simulink model "NE_Red_Rooster_Delta_B"  (R2016b)
settings: Solver=FixedStepAuto  StartTime=0.0  StopTime=inf  FixedStep=0.001  RelTol=1e-3
PreLoadFcn:
  | waijung.modelPreload; % Required for working with Waijung Blockset. Do not remove.
undefined symbols (not defined in the file): ARM, DiscIntNeverNeededParam, HSEOSC, Link, LQFP100, MDK, ST, STM32F407VG
libraries: simulink x20, stm32f4_io_lib x5, stm32f4_i2c_lib x4, stm32f4_reset_lib x1, stm32f4_device_config_lib x1
(part 2 of 3)

== system NE_Red_Rooster_Delta_B/Chart/sendpwm ==
  f : TriggerPort  TriggerType=function-call  VariantControl=Variant
      settings: CopyFcn=Stateflow.SLINSF.SimulinkMan.removeBlockPreDeleteFcn  PreDeleteFcn=Stateflow.SLINSF.SimulinkMan.unsafePredeleteFcn
  Data Store Read : DataStoreRead  DataStoreName=Left_Elevon
  Data Store Read1 : DataStoreRead  DataStoreName=Right_Elevon
  Data Store Read2 : DataStoreRead  DataStoreName=Throttle_Duty
  UART Tx3 : S-Function  Priority=1  FunctionName=stm32f4_usart  Parameters=configuration,uartmodule,transfer,baudrate,inputtype,outputtype,confstr,binheaderarray,binterminatorarray,asciiheader,asciiterminator,bindatalength,packetmode,varname,sampletime,sampletimestr,blockid  SFunctionDeploymentMode=off  EnableBusSupport=off  mask(stm32f4_usart){configuration=Tx, uartmodule=2, baudrate=115200, databits=8, parity=No, stopbit=1, remaptxpin=Not used, remaprxpin=Not used, flowcontrol=None, remapctspin=Not used, remaprtspin=Not used, advanceoptions=off, rxbuffersize=512, txbuffersize=512, transfer=Non-Blocking, packetmode=Binary, binheader='4F', binterminator='2E', porttype_double=0, porttype_single=3, porttype_int8=0, porttype_uint8=0, porttype_int16=0, porttype_uint16=0, porttype_int32=0, porttype_uint32=0, asciiformat='LE=%f, RE=%f, T=%f', rx_asciiterminator=CRLF (0x0D 0x0A - "\r\n"), tx_asciiterminator=CRLF (0x0D 0x0A - "\r\n"), storagename=<empty>, varname=, inputtype=[3  1 1 1], outputtype=[0], binheaderarray=[1 79], binterminatorarray=[1 46], bindatalength=12, asciiheader='LE=%f, RE=%f, T=%f\r\n', asciiterminator=[2 13 10], sampletime=-1, sampletimestr=-1, blockid=ChartsendpwmUARTTx3, confstr=[ "dummy", "0", "*", "*", "0", "*", "*", "0", "*", "*", "0", "*", "*", "1", "4", "6", "1", "4", "5", "512", "512", "1", "2", "115200", "8", "No", "1", "None", "USART2"], lastmodule=1}
      mask prompts: uartmodule "UART Module"; baudrate "Baud rate (bps)"; databits "Data bits"; stopbit "Stop bit"; remaptxpin "Tx Pin"; remaprxpin "Rx Pin"; flowcontrol "Hardware flow control"; remapctspin "HW Flow control, CTS Pin"; remaprtspin "HW Flow control, RTS Pin"; advanceoptions "Advance options"; rxbuffersize "Rx buffer size (bytes)"; txbuffersize "Tx buffer size (bytes)"; packetmode "Packet mode"; binheader "Binary header (example: '7E 7E')"; binterminator "Binary terminator (example: '03 03')"; porttype_double "Number of data port, type DOUBLE"; porttype_single "Number of data port, type SINGLE"; porttype_int8 "Number of data port, type INT8"; porttype_uint8 "Number of data port, type UINT8"; porttype_int16 "Number of data port, type INT16"; porttype_uint16 "Number of data port, type UINT16"; porttype_int32 "Number of data port, type INT32"; porttype_uint32 "Number of data port, type UINT32"; asciiformat "Ascii format"; rx_asciiterminator "End of packet"; tx_asciiterminator "End of packet"; storagename "Buffer"; varname "Var name"; inputtype "Input data type"; outputtype "Output data type"; binheaderarray "Binary header"; binterminatorarray "Binary terminator"; bindatalength "Binary data length"; asciiheader "Ascii header (printf format)"; asciiterminator "Ascii terminator"; sampletime "Sample time (sec)"; sampletimestr "Compiled sample time (sec) in string"; confstr "Configuration string"; lastmodule "Last module selected"
      mask help:
      | Data type for Ascii format
      | %u, %i, %d, %o, %x: uint32
      | %e, %g, %f: single
      | %c: int8
      mask init:
      | stm32f4_usart_callback('init');
      mask Help: web(fullfile(waijungdocroot,'stm32f4_usart_tx.htm'), '-browser')
      mask TypeOptions configuration: Setup | Tx | Rx
      mask Callback configuration: stm32f4_usart_callback('configuration');
      mask TypeOptions uartmodule: 1 | 2 | 3 | 4 | 5 | 6
      mask Callback uartmodule: stm32f4_usart_callback('uartmodule');
      mask Callback baudrate: stm32f4_usart_callback('baudrate');
      mask TypeOptions databits: 8
      mask TypeOptions parity: No | Odd | Even
      mask TypeOptions stopbit: 0.5 | 1 | 1.5 | 2
      mask TypeOptions remaptxpin: Not used | A9 | B6
      mask TypeOptions remaprxpin: Not used | A10 | B7
      mask TypeOptions flowcontrol: None | RTS | CTS | RTS/CTS
      mask Callback flowcontrol: stm32f4_usart_callback('flowcontrol');
      mask TypeOptions remapctspin: Not used | A11
      mask TypeOptions remaprtspin: Not used | A12
      mask Callback advanceoptions: stm32f4_usart_callback('advanceoptions');
      mask TypeOptions rxbuffersize: 16 | 32 | 64 | 128 | 256 | 512 | 1024 | 2048
      mask TypeOptions txbuffersize: 16 | 32 | 64 | 128 | 256 | 512 | 1024 | 2048
      mask TypeOptions transfer: Blocking | Non-Blocking
      mask Callback transfer: stm32f4_usart_callback('transfer');
      mask TypeOptions packetmode: Ascii | Binary | Binary Vector | String Buffer | Raw Buffer
      mask Callback packetmode: stm32f4_usart_callback('packetmode');
      mask Callback binheader: stm32f4_usart_callback('binheader');
      mask Callback binterminator: stm32f4_usart_callback('binterminator');
      mask Callback porttype_double: stm32f4_usart_callback('porttype');
      mask Callback porttype_single: stm32f4_usart_callback('porttype');
      mask Callback porttype_int8: stm32f4_usart_callback('porttype');
      mask Callback porttype_uint8: stm32f4_usart_callback('porttype');
      mask Callback porttype_int16: stm32f4_usart_callback('porttype');
      mask Callback porttype_uint16: stm32f4_usart_callback('porttype');
      mask Callback porttype_int32: stm32f4_usart_callback('porttype');
      mask Callback porttype_uint32: stm32f4_usart_callback('porttype');
      mask Callback asciiformat: stm32f4_usart_callback('asciiformat');
      mask TypeOptions rx_asciiterminator: CR (0x0D - "\r") | LF (0x0A - "\n") | CRLF (0x0D 0x0A - "\r\n")
      mask Callback rx_asciiterminator: stm32f4_usart_callback('rx_asciiterminator');
      mask TypeOptions tx_asciiterminator: CR (0x0D - "\r") | LF (0x0A - "\n") | CRLF (0x0D 0x0A - "\r\n") | None
      mask Callback tx_asciiterminator: stm32f4_usart_callback('tx_asciiterminator');
      mask TypeOptions storagename: <empty>
      mask Callback storagename: stm32f4_usart_callback('storagename');
      mask Callback varname: stm32f4_usart_callback('varname');
      mask Callback sampletime: stm32f4_usart_callback('sampletime');
      mask Callback sampletimestr: stm32f4_usart_callback('sampletimestr');
      mask Callback blockid: stm32f4_usart_callback('blockid');
      mask Display: text(0.5, 0.5, 'Module: USART2_Tx\nPacket: Binary\nTransfer: Non-Blocking\nTs (sec): -1','ver','middle','hor','center'); port_label('input', 1,'single'); port_label('input', 2,'single'); port_label('input', 3,'single');
  wires:
  Data Store Read2/1 -> UART Tx3/3
  Data Store Read1/1 -> UART Tx3/2
  Data Store Read/1 -> UART Tx3/1

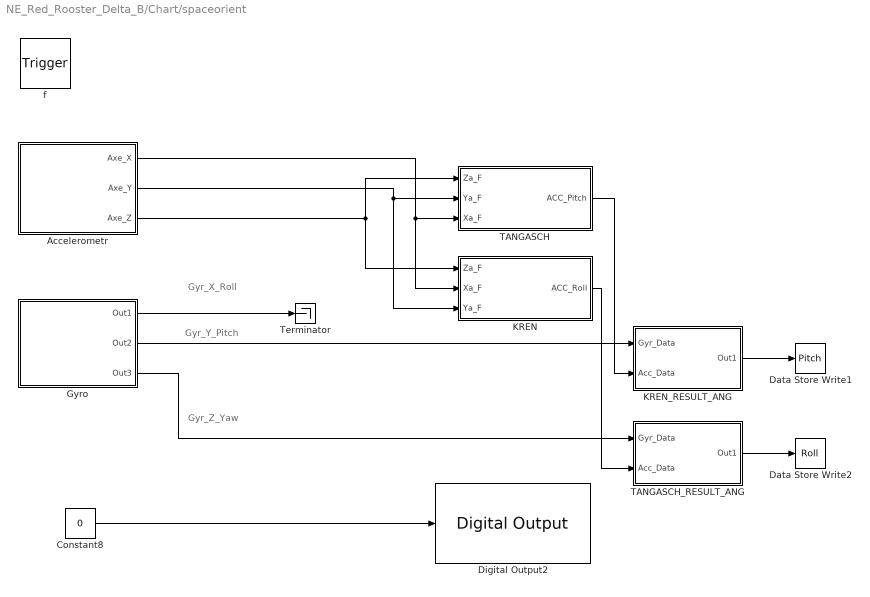
== system NE_Red_Rooster_Delta_B/Chart/spaceorient ==
  note: Gyr_X_Roll
  note: Gyr_Y_Pitch
  note: Gyr_Z_Yaw
  f : TriggerPort  TriggerType=function-call  VariantControl=Variant
      settings: CopyFcn=Stateflow.SLINSF.SimulinkMan.removeBlockPreDeleteFcn  PreDeleteFcn=Stateflow.SLINSF.SimulinkMan.unsafePredeleteFcn
  Accelerometr : Subsystem
      mask Display: image('ADXL345-1.jpg');
  Constant8 : Constant  Value=0
  Data Store Write1 : DataStoreWrite  DataStoreName=Pitch
  Data Store Write2 : DataStoreWrite  DataStoreName=Roll
  Digital Output2 : stm32f4_io_lib/Digital Output  use_bitband=on  port=D  speed=100  porttype=Push Pull  porttypestr=PP  use_pin0=off  use_pin1=off  use_pin2=off  use_pin3=off  use_pin4=off  use_pin5=off  use_pin6=off  use_pin7=off  use_pin8=off  use_pin9=off  use_pin10=off  use_pin11=off  use_pin12=off  use_pin13=off  use_pin14=off  use_pin15=on  pinstr=GPIO_Pin_15  usedpinarray="[0  0  0  0  0  0  0  0  0  0  0  0  0  0  0  1]"  bitbandingstr="#define ChartspaceorientDigitalOutput2_D15 Peripheral_BB(GPIOD->ODR, 15)  /* Output pin */"  sampletime=-1  sampletimestr=Inf  blockid=ChartspaceorientDigitalOutput2  enablecustomportlabel=off  globalinit=on  cinputportlabel=In1, In2  coutputportlabel=0
  Gyro : Subsystem
      mask Display: image('L3GD20H.jpg');
  KREN : Subsystem
  KREN_RESULT_ANG : Subsystem
  TANGASCH : Subsystem
  TANGASCH_RESULT_ANG : Subsystem
  Terminator : Terminator
  wires:
  Gyro/1(Out1) -> Terminator/1
  Accelerometr/1(Axe_X) -> TANGASCH/3(Xa_F), KREN/2(Xa_F)
  Accelerometr/2(Axe_Y) -> KREN/3(Ya_F), TANGASCH/2(Ya_F)
  Accelerometr/3(Axe_Z) -> KREN/1(Za_F), TANGASCH/1(Za_F)
  Gyro/3(Out3) -> TANGASCH_RESULT_ANG/1(Gyr_Data)
  Gyro/2(Out2) -> KREN_RESULT_ANG/1(Gyr_Data)
  TANGASCH/1(ACC_Pitch) -> KREN_RESULT_ANG/2(Acc_Data)
  KREN/1(ACC_Roll) -> TANGASCH_RESULT_ANG/2(Acc_Data)
  KREN_RESULT_ANG/1(Out1) -> Data Store Write1/1
  TANGASCH_RESULT_ANG/1(Out1) -> Data Store Write2/1
  Constant8/1 -> Digital Output2/1

== system NE_Red_Rooster_Delta_B/Reset_Subsystem ==
  Compare To Constant : simulink/Logic and Bit Operations/Compare To Constant  relop===  const=1.0  OutDataTypeStr=boolean
  Digital Input : stm32f4_io_lib/Digital Input  port=A  speed=100  porttype=None  porttypestr=NOPULL  use_pin0=on  use_pin1=off  use_pin2=off  use_pin3=off  use_pin4=off  use_pin5=off  use_pin6=off  use_pin7=off  use_pin8=off  use_pin9=off  use_pin10=off  use_pin11=off  use_pin12=off  use_pin13=off  use_pin14=off  use_pin15=off  pinstr=GPIO_Pin_0  usedpinarray="[1  0  0  0  0  0  0  0  0  0  0  0  0  0  0  0]"  bitbandingstr="#define Reset_SubsystemDigitalInput_A0 Peripheral_BB(GPIOA->IDR, 0)  /* Output pin */"  sampletime=-1  sampletimestr=0.01  blockid=Reset_SubsystemDigitalInput  enablecustomportlabel=off  glabalinit=off  cinputportlabel=In1, In2  coutputportlabel=Out1, Out2
  Enabled Subsystem : Subsystem  TreatAsAtomicUnit=on
  wires:
  Compare To Constant/1 -> Enabled Subsystem/Enable
  Digital Input/1 -> Compare To Constant/1

== system NE_Red_Rooster_Delta_B/Chart/initaccel/Init_ADXL345 ==
  Enable : EnablePort
  Compare To Zero : simulink/Logic and Bit Operations/Compare To Zero  relop===  OutDataTypeStr=boolean
  Constant : Constant  Value=0
  Constant1 : Constant  Value=hex2dec('A6')  OutDataTypeStr=uint8  SampleTime=-1
  Constant8 : Constant  Value=hex2dec('2D')  OutDataTypeStr=uint8  SampleTime=-1
  Constant9 : Constant  Value=hex2dec('08')  OutDataTypeStr=uint8  SampleTime=-1
  Data Store Write : DataStoreWrite  DataStoreName=Init_ADXL
  Digital Output1 : stm32f4_io_lib/Digital Output  use_bitband=on  port=D  speed=100  porttype=Push Pull  porttypestr=PP  use_pin0=off  use_pin1=off  use_pin2=off  use_pin3=off  use_pin4=off  use_pin5=off  use_pin6=off  use_pin7=off  use_pin8=off  use_pin9=off  use_pin10=off  use_pin11=off  use_pin12=off  use_pin13=on  use_pin14=off  use_pin15=off  pinstr=GPIO_Pin_13  usedpinarray="[0  0  0  0  0  0  0  0  0  0  0  0  0  1  0  0]"  bitbandingstr="#define ChartinitaccelInit_ADXL345DigitalOutput1_D13 Peripheral_BB(GPIOD->ODR, 13)  /* Output pin */"  sampletime=-1  sampletimestr=Inf  blockid=ChartinitaccelInit_ADXL345DigitalOutput1  enablecustomportlabel=off  globalinit=off  cinputportlabel=In1, In2  coutputportlabel=0
  I2C Master Read/Write1 : stm32f4_i2c_lib/I2C Master Read//Write  configuration=Transaction  module=1  lastmodule=3  transfer=Blocking  dutycycle=TLow/THigh = 2  clkspeed=400  timeout=25  writecount=2  readcount=0  sdapin=C9  sclpin=A8  waitwritetime=0  forcestop=off  inputtypearray=[3 3 3 3]  outputtypearray=[1 3]  confstr="[\"C\",\"9\",\"A\",\"8\",\"1\",\"1\",\"6\",\"0\",\"I2C_DutyCycle_2\",\"0\",\"off\"]"  sampletime=-1  sampletimestr=-1  blockid=ChartinitaccelInit_ADXL345I2CMasterReadWrite1
  Subsystem : Subsystem
  Terminator : Terminator
  wires:
  Constant9/1 -> I2C Master Read/Write1/3
  I2C Master Read/Write1/1 -> Compare To Zero/1
  Constant1/1 -> I2C Master Read/Write1/1
  Constant8/1 -> I2C Master Read/Write1/2
  Compare To Zero/1 -> Subsystem/Enable
  Subsystem/1(Out1) -> Terminator/1
  Constant/1 -> Digital Output1/1, Data Store Write/1

== system NE_Red_Rooster_Delta_B/Chart/initgyro/Init_L3GD4200  ==
  Enable : EnablePort
  Compare To Zero : simulink/Logic and Bit Operations/Compare To Zero  relop===  OutDataTypeStr=boolean  ZeroCross=off
  Constant : Constant  Value=0
  Data Store Write : DataStoreWrite  DataStoreName=Init_L3GD
  Get Init L3G4200D1 : Subsystem
  Init L3G4200D : Subsystem  TreatAsAtomicUnit=on
  SlvAddr1 : Constant  Value=hex2dec('D2')  OutDataTypeStr=uint8  SampleTime=-1
  wires:
  Compare To Zero/1 -> Init L3G4200D/Enable
  Get Init L3G4200D1/1(Initial Done) -> Compare To Zero/1
  SlvAddr1/1 -> Get Init L3G4200D1/1(SlvAddr)
  Constant/1 -> Data Store Write/1

== system NE_Red_Rooster_Delta_B/Chart/pwm/If Action Subsystem ==
  In1 : Inport
  In2 : Inport  Port=2
  In3 : Inport  Port=3
  Action Port : ActionPort  ActionType=then
  Out1 : Outport
  Out2 : Outport  Port=2
  Out3 : Outport  Port=3
  wires:
  In1/1 -> Out1/1
  In2/1 -> Out2/1
  In3/1 -> Out3/1

== system NE_Red_Rooster_Delta_B/Chart/pwm/If Action Subsystem1 ==
  In1 : Inport
  In2 : Inport  Port=2
  In3 : Inport  Port=3
  Action Port : ActionPort  ActionType=then
  Out1 : Outport
  Out2 : Outport  Port=2
  Out3 : Outport  Port=3
  wires:
  In1/1 -> Out1/1
  In2/1 -> Out2/1
  In3/1 -> Out3/1

== system NE_Red_Rooster_Delta_B/Chart/pwm/If Action Subsystem2 ==
  In1 : Inport
  In2 : Inport  Port=2
  In3 : Inport  Port=3
  Action Port : ActionPort  ActionType=then
  Out1 : Outport
  Out2 : Outport  Port=2
  Out3 : Outport  Port=3
  wires:
  In3/1 -> Out3/1
  In2/1 -> Out2/1
  In1/1 -> Out1/1

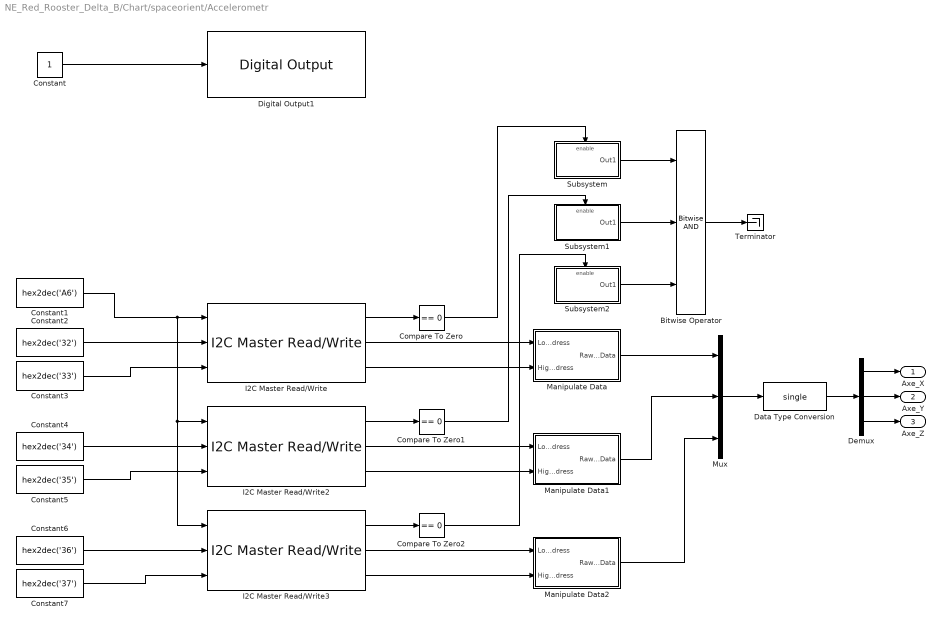
== system NE_Red_Rooster_Delta_B/Chart/spaceorient/Accelerometr ==
  Bitwise Operator : simulink/Logic and Bit Operations/Bitwise Operator  logicop=AND  UseBitMask=off  NumInputPorts=3  BitMask=bin2dec('11011001')  BitMaskRealWorld=Stored Integer
  Compare To Zero : simulink/Logic and Bit Operations/Compare To Zero  relop===  OutDataTypeStr=boolean
  Compare To Zero1 : simulink/Logic and Bit Operations/Compare To Zero  relop===  OutDataTypeStr=boolean
  Compare To Zero2 : simulink/Logic and Bit Operations/Compare To Zero  relop===  OutDataTypeStr=boolean
  Constant : Constant
  Constant1 : Constant  Value=hex2dec('A6')  OutDataTypeStr=uint8  SampleTime=-1
  Constant2 : Constant  Value=hex2dec('32')  OutDataTypeStr=uint8  SampleTime=-1
  Constant3 : Constant  Value=hex2dec('33')  OutDataTypeStr=uint8  SampleTime=-1
  Constant4 : Constant  Value=hex2dec('34')  OutDataTypeStr=uint8  SampleTime=-1
  Constant5 : Constant  Value=hex2dec('35')  OutDataTypeStr=uint8  SampleTime=-1
  Constant6 : Constant  Value=hex2dec('36')  OutDataTypeStr=uint8  SampleTime=-1
  Constant7 : Constant  Value=hex2dec('37')  OutDataTypeStr=uint8  SampleTime=-1
  Data Type Conversion : DataTypeConversion  OutDataTypeStr=single
  Demux : Demux  Outputs=3
  Digital Output1 : stm32f4_io_lib/Digital Output  use_bitband=on  port=D  speed=100  porttype=Push Pull  porttypestr=PP  use_pin0=off  use_pin1=off  use_pin2=off  use_pin3=off  use_pin4=off  use_pin5=off  use_pin6=off  use_pin7=off  use_pin8=off  use_pin9=off  use_pin10=off  use_pin11=off  use_pin12=off  use_pin13=off  use_pin14=off  use_pin15=on  pinstr=GPIO_Pin_15  usedpinarray="[0  0  0  0  0  0  0  0  0  0  0  0  0  0  0  1]"  bitbandingstr="#define ChartspaceorientAccelerometrDigitalOutput1_D15 Peripheral_BB(GPIOD->ODR, 15)  /* Output pin */"  sampletime=-1  sampletimestr=Inf  blockid=ChartspaceorientAccelerometrDigitalOutput1  enablecustomportlabel=off  globalinit=on  cinputportlabel=In1, In2  coutputportlabel=0
  I2C Master Read/Write : stm32f4_i2c_lib/I2C Master Read//Write  configuration=Transaction  module=1  lastmodule=3  transfer=Blocking  dutycycle=TLow/THigh = 2  clkspeed=400  timeout=25  writecount=2  readcount=2  sdapin=C9  sclpin=A8  waitwritetime=0  forcestop=off  inputtypearray=[3 3 3 3]  outputtypearray=[3 3 3 3]  confstr="[\"C\",\"9\",\"A\",\"8\",\"1\",\"1\",\"6\",\"0\",\"I2C_DutyCycle_2\",\"0\",\"off\"]"  sampletime=-1  sampletimestr=-1  blockid=ChartspaceorientAccelerometrI2CMasterReadWrite
  I2C Master Read/Write2 : stm32f4_i2c_lib/I2C Master Read//Write  configuration=Transaction  module=1  lastmodule=3  transfer=Blocking  dutycycle=TLow/THigh = 2  clkspeed=400  timeout=25  writecount=2  readcount=2  sdapin=C9  sclpin=A8  waitwritetime=0  forcestop=off  inputtypearray=[3 3 3 3]  outputtypearray=[3 3 3 3]  confstr="[\"C\",\"9\",\"A\",\"8\",\"1\",\"1\",\"6\",\"0\",\"I2C_DutyCycle_2\",\"0\",\"off\"]"  sampletime=-1  sampletimestr=-1  blockid=ChartspaceorientAccelerometrI2CMasterReadWrite2
  I2C Master Read/Write3 : stm32f4_i2c_lib/I2C Master Read//Write  configuration=Transaction  module=1  lastmodule=3  transfer=Blocking  dutycycle=TLow/THigh = 2  clkspeed=400  timeout=25  writecount=2  readcount=2  sdapin=C9  sclpin=A8  waitwritetime=0  forcestop=off  inputtypearray=[3 3 3 3]  outputtypearray=[3 3 3 3]  confstr="[\"C\",\"9\",\"A\",\"8\",\"1\",\"1\",\"6\",\"0\",\"I2C_DutyCycle_2\",\"0\",\"off\"]"  sampletime=-1  sampletimestr=-1  blockid=ChartspaceorientAccelerometrI2CMasterReadWrite3
  Manipulate Data : Subsystem
  Manipulate Data1 : Subsystem
  Manipulate Data2 : Subsystem
  Mux : Mux  Inputs=3
  Subsystem : Subsystem
  Subsystem1 : Subsystem
  Subsystem2 : Subsystem
  Terminator : Terminator
  Axe_X : Outport
  Axe_Y : Outport  Port=2
  Axe_Z : Outport  Port=3
  wires:
  I2C Master Read/Write3/2 -> Manipulate Data2/1(LowAddress)
  I2C Master Read/Write2/3 -> Manipulate Data1/2(HighAddress)
  I2C Master Read/Write/1 -> Compare To Zero/1
  Constant7/1 -> I2C Master Read/Write3/3
  I2C Master Read/Write3/3 -> Manipulate Data2/2(HighAddress)
  Mux/1 -> Data Type Conversion/1
  Constant4/1 -> I2C Master Read/Write2/2
  Constant1/1 -> I2C Master Read/Write3/1, I2C Master Read/Write2/1, I2C Master Read/Write/1
  I2C Master Read/Write2/2 -> Manipulate Data1/1(LowAddress)
  I2C Master Read/Write/3 -> Manipulate Data/2(HighAddress)
  I2C Master Read/Write3/1 -> Compare To Zero2/1
  Constant6/1 -> I2C Master Read/Write3/2
  Manipulate Data2/1(RawAccData) -> Mux/3
  Constant5/1 -> I2C Master Read/Write2/3
  Manipulate Data1/1(RawAccData) -> Mux/2
  I2C Master Read/Write/2 -> Manipulate Data/1(LowAddress)
  Constant2/1 -> I2C Master Read/Write/2
  Constant3/1 -> I2C Master Read/Write/3
  I2C Master Read/Write2/1 -> Compare To Zero1/1
  Manipulate Data/1(RawAccData) -> Mux/1
  Compare To Zero/1 -> Subsystem/Enable
  Compare To Zero1/1 -> Subsystem1/Enable
  Compare To Zero2/1 -> Subsystem2/Enable
  Data Type Conversion/1 -> Demux/1
  Demux/2 -> Axe_Y/1
  Demux/1 -> Axe_X/1
  Demux/3 -> Axe_Z/1
  Subsystem/1(Out1) -> Bitwise Operator/1
  Subsystem1/1(Out1) -> Bitwise Operator/2
  Subsystem2/1(Out1) -> Bitwise Operator/3
  Bitwise Operator/1 -> Terminator/1
  Constant/1 -> Digital Output1/1

== system NE_Red_Rooster_Delta_B/Chart/spaceorient/Gyro ==
  Compare To Zero1 : simulink/Logic and Bit Operations/Compare To Zero  relop===  OutDataTypeStr=boolean  ZeroCross=off
  Data_transformation : Subsystem
  L3G4200D : Subsystem
  Success : Subsystem
      mask Display: image('C:\Users\Alexander Gorbunov\Pictures\Roll_Pitch_Yaw.JPG');
  Out1 : Outport
  Out2 : Outport  Port=2
  Out3 : Outport  Port=3
  wires:
  Success/1(Gyr_X) -> Data_transformation/1(In1)
  L3G4200D/1(Status) -> Compare To Zero1/1
  L3G4200D/4(Z) -> Success/3(In3)
  L3G4200D/3(Y) -> Success/2(In2)
  Success/2(Gyr_Y) -> Data_transformation/2(In2)
  Success/3(Gyr_Z) -> Data_transformation/3(In3)
  L3G4200D/2(X) -> Success/1(In1)
  Compare To Zero1/1 -> Success/Enable
  Data_transformation/1(Out1) -> Out1/1
  Data_transformation/2(Out2) -> Out2/1
  Data_transformation/3(Out3) -> Out3/1

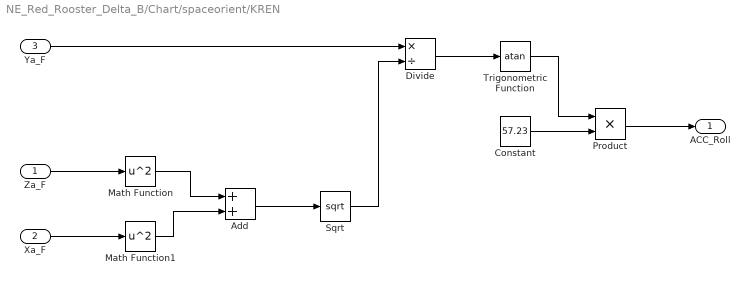
== system NE_Red_Rooster_Delta_B/Chart/spaceorient/KREN ==
  Za_F : Inport
  Xa_F : Inport  Port=2
  Ya_F : Inport  Port=3
  Add : Sum
  Constant : Constant  Value=57.23
  Divide : Product  Inputs=*/
  Math Function : Math  Operator=square  SaturateOnIntegerOverflow=on
  Math Function1 : Math  Operator=square  SaturateOnIntegerOverflow=on
  Product : Product
  Sqrt : Sqrt  SaturateOnIntegerOverflow=on
  Trigonometric Function : Trigonometry  Operator=atan
  ACC_Roll : Outport
  wires:
  Sqrt/1 -> Divide/2
  Za_F/1 -> Math Function/1
  Ya_F/1 -> Divide/1
  Xa_F/1 -> Math Function1/1
  Add/1 -> Sqrt/1
  Trigonometric Function/1 -> Product/1
  Divide/1 -> Trigonometric Function/1
  Math Function/1 -> Add/1
  Math Function1/1 -> Add/2
  Constant/1 -> Product/2
  Product/1 -> ACC_Roll/1

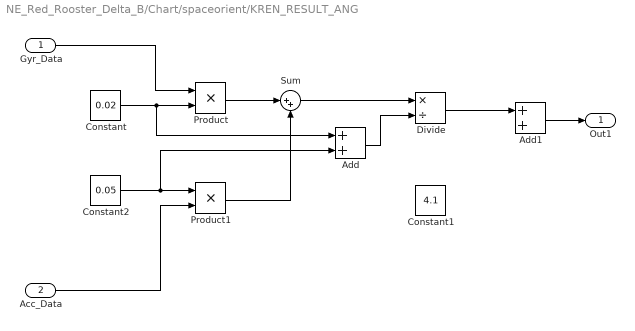
== system NE_Red_Rooster_Delta_B/Chart/spaceorient/KREN_RESULT_ANG ==
  Gyr_Data : Inport
  Acc_Data : Inport  Port=2
  Add : Sum
  Add1 : Sum
  Constant : Constant  Value=0.02
  Constant1 : Constant  Value=4.1
  Constant2 : Constant  Value=0.05
  Divide : Product  Inputs=*/
  Product : Product
  Product1 : Product
  Sum : Sum  Inputs=|++
  Out1 : Outport
  wires:
  Acc_Data/1 -> Product1/2
  Constant/1 -> Add/1, Product/2
  Product/1 -> Sum/1
  Product1/1 -> Sum/2
  Constant2/1 -> Add/2, Product1/1
  Gyr_Data/1 -> Product/1
  Sum/1 -> Divide/1
  Add/1 -> Divide/2
  Divide/1 -> Add1/1
  Add1/1 -> Out1/1

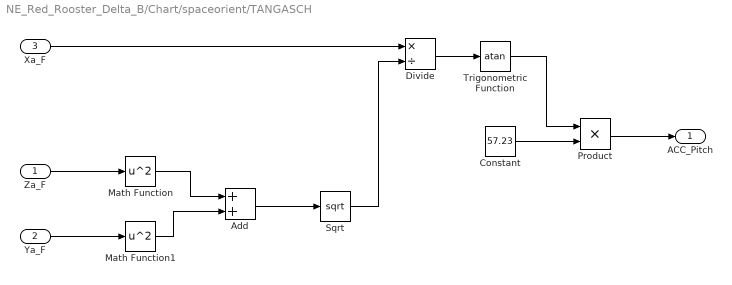
== system NE_Red_Rooster_Delta_B/Chart/spaceorient/TANGASCH ==
  Za_F : Inport
  Ya_F : Inport  Port=2
  Xa_F : Inport  Port=3
  Add : Sum
  Constant : Constant  Value=57.23
  Divide : Product  Inputs=*/
  Math Function : Math  Operator=square  SaturateOnIntegerOverflow=on
  Math Function1 : Math  Operator=square  SaturateOnIntegerOverflow=on
  Product : Product
  Sqrt : Sqrt  SaturateOnIntegerOverflow=on
  Trigonometric Function : Trigonometry  Operator=atan
  ACC_Pitch : Outport
  wires:
  Math Function1/1 -> Add/2
  Math Function/1 -> Add/1
  Divide/1 -> Trigonometric Function/1
  Trigonometric Function/1 -> Product/1
  Add/1 -> Sqrt/1
  Ya_F/1 -> Math Function1/1
  Xa_F/1 -> Divide/1
  Za_F/1 -> Math Function/1
  Sqrt/1 -> Divide/2
  Constant/1 -> Product/2
  Product/1 -> ACC_Pitch/1

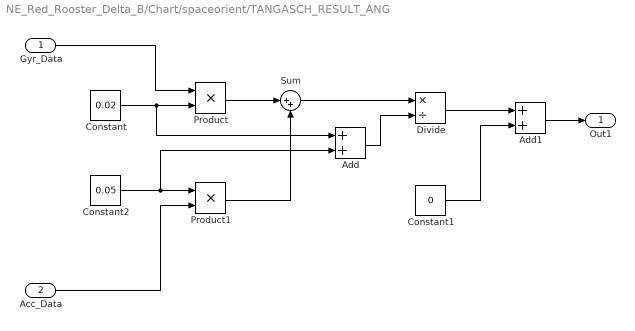
== system NE_Red_Rooster_Delta_B/Chart/spaceorient/TANGASCH_RESULT_ANG ==
  Gyr_Data : Inport
  Acc_Data : Inport  Port=2
  Add : Sum
  Add1 : Sum
  Constant : Constant  Value=0.02
  Constant1 : Constant  Value=0
  Constant2 : Constant  Value=0.05
  Divide : Product  Inputs=*/
  Product : Product
  Product1 : Product
  Sum : Sum  Inputs=|++
  Out1 : Outport
  wires:
  Constant1/1 -> Add1/2
  Add1/1 -> Out1/1
  Divide/1 -> Add1/1
  Add/1 -> Divide/2
  Sum/1 -> Divide/1
  Gyr_Data/1 -> Product/1
  Constant2/1 -> Product1/1, Add/2
  Product1/1 -> Sum/2
  Product/1 -> Sum/1
  Constant/1 -> Product/2, Add/1
  Acc_Data/1 -> Product1/2

== system NE_Red_Rooster_Delta_B/Reset_Subsystem/Enabled Subsystem ==
  Enable : EnablePort
  System Reset : stm32f4_reset_lib/System Reset  conf=<empty>  sampletime=-1  sampletimestr=0.01  blockid=Reset_SubsystemEnabledSubsystemSystemReset  inputarray=[]  inputlabelarray={}  outputarray=[]  outputlabelarray={}  compat=0  confstr="[\"Param1\",\"Param1\"]"

== system NE_Red_Rooster_Delta_B/Chart/initaccel/Init_ADXL345/Subsystem ==
  Enable : EnablePort
  Constant : Constant
  Out1 : Outport
  wires:
  Constant/1 -> Out1/1

== system NE_Red_Rooster_Delta_B/Chart/initgyro/Init_L3GD4200 /Get Init L3G4200D1 ==
  SlvAddr : Inport
  Bitwise Operator : simulink/Logic and Bit Operations/Bitwise Operator  logicop=AND  UseBitMask=off  NumInputPorts=4  BitMask=bin2dec('11011001')  BitMaskRealWorld=Stored Integer
  CNTRL_REG1 : Constant  Value=hex2dec('20')  OutDataTypeStr=uint8  SampleTime=-1
  CNTRL_REG4 : Constant  Value=hex2dec('23')  OutDataTypeStr=uint8  SampleTime=-1
  Compare To Constant : simulink/Logic and Bit Operations/Compare To Constant  relop===  const=0  OutDataTypeStr=uint8  ZeroCross=off
  Compare To Constant1 : simulink/Logic and Bit Operations/Compare To Constant  relop===  const=hex2dec('0F')  OutDataTypeStr=uint8  ZeroCross=off
  Compare To Constant2 : simulink/Logic and Bit Operations/Compare To Constant  relop===  const=0  OutDataTypeStr=uint8  ZeroCross=off
  Compare To Constant3 : simulink/Logic and Bit Operations/Compare To Constant  relop===  const=0  OutDataTypeStr=uint8  ZeroCross=off
  I2C Master Read/Write : S-Function  FunctionName=stm32f4_i2c  Parameters=configuration,module,transfer,clkspeed,timeout,sdapin,sclpin,writecount,readcount,inputtypearray,outputtypearray,confstr,sampletime,sampletimestr,blockid  SFunctionDeploymentMode=off  EnableBusSupport=off  mask(stm32f4_i2c){configuration=Transaction, module=1, lastmodule=3, transfer=Blocking, dutycycle=TLow/THigh = 2, clkspeed=400, timeout=25, writecount=1, readcount=1, sdapin=C9, sclpin=A8, waitwritetime=0, inputtypearray=[2 3 3], outputtypearray=[2 3 3], confstr=["C","9","A","8","1","1","6","0","I2C_DutyCycle_2","0","off"], sampletime=-1, sampletimestr=-1, blockid=ChartinitgyroInit_L3GD4200GetInitL3G4200D1I2CMasterReadWrite}
      mask prompts: module "I2C Module"; lastmodule "Last module"; transfer "Transfer mode"; dutycycle "Duty cycle in fast mode"; clkspeed "Clock speed (kHz)"; timeout "Timeout (ms)"; writecount "Bytes write count"; readcount "Bytes read count"; sdapin "SDA pin"; sclpin "SCL pin"; waitwritetime "Wait write time (ms), default is 0"; inputtypearray "Input type array"; outputtypearray "Output type array"; confstr "Configuration string"; sampletime "Sample time (sec)"; sampletimestr "Compiled sample time (sec) in string"
      mask init:
      | stm32f4_i2c_callback('init');
      mask Help: web(fullfile(waijungdocroot,'stm32f4_i2c.htm'), '-browser')
      mask TypeOptions configuration: Setup | Transaction
      mask Callback configuration: stm32f4_i2c_callback('configuration');
      mask TypeOptions module: 1 | 2 | 3
      mask Callback module: stm32f4_i2c_callback('module');
      mask TypeOptions transfer: Blocking | Non-blocking
      mask TypeOptions dutycycle: TLow/THigh = 16/9 | TLow/THigh = 2
      mask Callback dutycycle: stm32f4_i2c_callback('dutycycle');
      mask Callback writecount: stm32f4_i2c_callback('writecount');
      mask Callback readcount: stm32f4_i2c_callback('readcount');
      mask TypeOptions sdapin: - | C9
      mask Callback sdapin: stm32f4_i2c_callback('sdapin');
      mask TypeOptions sclpin: - | A8
      mask Callback sclpin: stm32f4_i2c_callback('sclpin');
      mask Callback confstr: stm32f4_i2c_callback('confstr');
      mask Callback sampletime: stm32f4_i2c_callback('sampletime');
      mask Callback sampletimestr: stm32f4_i2c_callback('sampletimestr');
      mask Callback blockid: stm32f4_i2c_callback('blockid');
      mask Display: text(0.5, 0.5, 'Module: I2C1\nTransfer: Blocking\nWrite: 1 bytes\nRead: 1 bytes\nTs (sec): -1','ver','middle','hor','center');port_label('input', 1,'SlvAddr');port_label('input', 2,'Wr0 (uint8)');port_label('output', 1,'Status');port_label('output', 2,'Rd0 (uint8)');
  I2C Master Read/Write1 : S-Function  FunctionName=stm32f4_i2c  Parameters=configuration,module,transfer,clkspeed,timeout,sdapin,sclpin,writecount,readcount,inputtypearray,outputtypearray,confstr,sampletime,sampletimestr,blockid  SFunctionDeploymentMode=off  EnableBusSupport=off  mask(stm32f4_i2c){configuration=Transaction, module=1, lastmodule=3, transfer=Blocking, dutycycle=TLow/THigh = 2, clkspeed=400, timeout=25, writecount=1, readcount=1, sdapin=C9, sclpin=A8, waitwritetime=0, inputtypearray=[2 3 3], outputtypearray=[2 3 3], confstr=["C","9","A","8","1","1","6","0","I2C_DutyCycle_2","0","off"], sampletime=-1, sampletimestr=-1, blockid=ChartinitgyroInit_L3GD4200GetInitL3G4200D1I2CMasterReadWrite1}
      mask prompts: module "I2C Module"; lastmodule "Last module"; transfer "Transfer mode"; dutycycle "Duty cycle in fast mode"; clkspeed "Clock speed (kHz)"; timeout "Timeout (ms)"; writecount "Bytes write count"; readcount "Bytes read count"; sdapin "SDA pin"; sclpin "SCL pin"; waitwritetime "Wait write time (ms), default is 0"; inputtypearray "Input type array"; outputtypearray "Output type array"; confstr "Configuration string"; sampletime "Sample time (sec)"; sampletimestr "Compiled sample time (sec) in string"
      mask init:
      | stm32f4_i2c_callback('init');
      mask Help: web(fullfile(waijungdocroot,'stm32f4_i2c.htm'), '-browser')
      mask TypeOptions configuration: Setup | Transaction
      mask Callback configuration: stm32f4_i2c_callback('configuration');
      mask TypeOptions module: 1 | 2 | 3
      mask Callback module: stm32f4_i2c_callback('module');
      mask TypeOptions transfer: Blocking | Non-blocking
      mask TypeOptions dutycycle: TLow/THigh = 16/9 | TLow/THigh = 2
      mask Callback dutycycle: stm32f4_i2c_callback('dutycycle');
      mask Callback writecount: stm32f4_i2c_callback('writecount');
      mask Callback readcount: stm32f4_i2c_callback('readcount');
      mask TypeOptions sdapin: - | C9
      mask Callback sdapin: stm32f4_i2c_callback('sdapin');
      mask TypeOptions sclpin: - | A8
      mask Callback sclpin: stm32f4_i2c_callback('sclpin');
      mask Callback confstr: stm32f4_i2c_callback('confstr');
      mask Callback sampletime: stm32f4_i2c_callback('sampletime');
      mask Callback sampletimestr: stm32f4_i2c_callback('sampletimestr');
      mask Callback blockid: stm32f4_i2c_callback('blockid');
      mask Display: text(0.5, 0.5, 'Module: I2C1\nTransfer: Blocking\nWrite: 1 bytes\nRead: 1 bytes\nTs (sec): -1','ver','middle','hor','center');port_label('input', 1,'SlvAddr');port_label('input', 2,'Wr0 (uint8)');port_label('output', 1,'Status');port_label('output', 2,'Rd0 (uint8)');
  Initial Done : Outport
  wires:
  Compare To Constant3/1 -> Bitwise Operator/4
  Compare To Constant2/1 -> Bitwise Operator/3
  Compare To Constant1/1 -> Bitwise Operator/2
  Compare To Constant/1 -> Bitwise Operator/1
  Bitwise Operator/1 -> Initial Done/1
  I2C Master Read/Write1/2 -> Compare To Constant3/1
  I2C Master Read/Write1/1 -> Compare To Constant2/1
  I2C Master Read/Write/2 -> Compare To Constant1/1
  I2C Master Read/Write/1 -> Compare To Constant/1
  SlvAddr/1 -> I2C Master Read/Write/1, I2C Master Read/Write1/1
  CNTRL_REG1/1 -> I2C Master Read/Write/2
  CNTRL_REG4/1 -> I2C Master Read/Write1/2

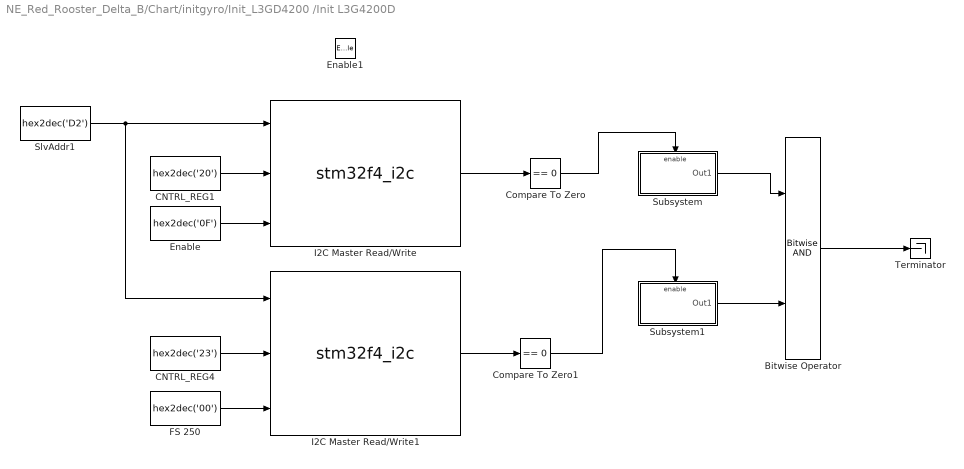
== system NE_Red_Rooster_Delta_B/Chart/initgyro/Init_L3GD4200 /Init L3G4200D ==
  Enable1 : EnablePort  PropagateVarSize=During execution
  Bitwise Operator : simulink/Logic and Bit Operations/Bitwise Operator  logicop=AND  UseBitMask=off  NumInputPorts=2  BitMask=bin2dec('11011001')  BitMaskRealWorld=Stored Integer
  CNTRL_REG1 : Constant  Value=hex2dec('20')  OutDataTypeStr=uint8  SampleTime=-1
  CNTRL_REG4 : Constant  Value=hex2dec('23')  OutDataTypeStr=uint8  SampleTime=-1
  Compare To Zero : simulink/Logic and Bit Operations/Compare To Zero  relop===  OutDataTypeStr=boolean
  Compare To Zero1 : simulink/Logic and Bit Operations/Compare To Zero  relop===  OutDataTypeStr=boolean
  Enable : Constant  Value=hex2dec('0F')  OutDataTypeStr=uint8  SampleTime=-1
  FS 250 : Constant  Value=hex2dec('00')  OutDataTypeStr=uint8  SampleTime=-1
  I2C Master Read/Write : S-Function  FunctionName=stm32f4_i2c  Parameters=configuration,module,transfer,clkspeed,timeout,sdapin,sclpin,writecount,readcount,inputtypearray,outputtypearray,confstr,sampletime,sampletimestr,blockid  SFunctionDeploymentMode=off  EnableBusSupport=off  mask(stm32f4_i2c){configuration=Transaction, module=1, lastmodule=3, transfer=Blocking, dutycycle=TLow/THigh = 2, clkspeed=400, timeout=25, writecount=2, readcount=0, sdapin=C9, sclpin=A8, waitwritetime=0, inputtypearray=[3 3 3 3], outputtypearray=[1 3], confstr=["C","9","A","8","1","1","6","0","I2C_DutyCycle_2","0","off"], sampletime=-1, sampletimestr=-1, blockid=ChartinitgyroInit_L3GD4200InitL3G4200DI2CMasterReadWrite}
      mask prompts: module "I2C Module"; lastmodule "Last module"; transfer "Transfer mode"; dutycycle "Duty cycle in fast mode"; clkspeed "Clock speed (kHz)"; timeout "Timeout (ms)"; writecount "Bytes write count"; readcount "Bytes read count"; sdapin "SDA pin"; sclpin "SCL pin"; waitwritetime "Wait write time (ms), default is 0"; inputtypearray "Input type array"; outputtypearray "Output type array"; confstr "Configuration string"; sampletime "Sample time (sec)"; sampletimestr "Compiled sample time (sec) in string"
      mask init:
      | stm32f4_i2c_callback('init');
      mask Help: web(fullfile(waijungdocroot,'stm32f4_i2c.htm'), '-browser')
      mask TypeOptions configuration: Setup | Transaction
      mask Callback configuration: stm32f4_i2c_callback('configuration');
      mask TypeOptions module: 1 | 2 | 3
      mask Callback module: stm32f4_i2c_callback('module');
      mask TypeOptions transfer: Blocking | Non-blocking
      mask TypeOptions dutycycle: TLow/THigh = 16/9 | TLow/THigh = 2
      mask Callback dutycycle: stm32f4_i2c_callback('dutycycle');
      mask Callback writecount: stm32f4_i2c_callback('writecount');
      mask Callback readcount: stm32f4_i2c_callback('readcount');
      mask TypeOptions sdapin: - | C9
      mask Callback sdapin: stm32f4_i2c_callback('sdapin');
      mask TypeOptions sclpin: - | A8
      mask Callback sclpin: stm32f4_i2c_callback('sclpin');
      mask Callback confstr: stm32f4_i2c_callback('confstr');
      mask Callback sampletime: stm32f4_i2c_callback('sampletime');
      mask Callback sampletimestr: stm32f4_i2c_callback('sampletimestr');
      mask Callback blockid: stm32f4_i2c_callback('blockid');
      mask Display: text(0.5, 0.5, 'Module: I2C1\nTransfer: Blocking\nWrite: 2 bytes\nRead: 0 bytes\nTs (sec): -1','ver','middle','hor','center');port_label('input', 1,'SlvAddr');port_label('input', 2,'Wr0 (uint8)');port_label('input', 3,'Wr1 (uint8)');port_label('output', 1,'Status');
  I2C Master Read/Write1 : S-Function  FunctionName=stm32f4_i2c  Parameters=configuration,module,transfer,clkspeed,timeout,sdapin,sclpin,writecount,readcount,inputtypearray,outputtypearray,confstr,sampletime,sampletimestr,blockid  SFunctionDeploymentMode=off  EnableBusSupport=off  mask(stm32f4_i2c){configuration=Transaction, module=1, lastmodule=3, transfer=Blocking, dutycycle=TLow/THigh = 2, clkspeed=400, timeout=25, writecount=2, readcount=0, sdapin=C9, sclpin=A8, waitwritetime=0, inputtypearray=[3 3 3 3], outputtypearray=[1 3], confstr=["C","9","A","8","1","1","6","0","I2C_DutyCycle_2","0","off"], sampletime=-1, sampletimestr=-1, blockid=ChartinitgyroInit_L3GD4200InitL3G4200DI2CMasterReadWrite1}
      mask prompts: module "I2C Module"; lastmodule "Last module"; transfer "Transfer mode"; dutycycle "Duty cycle in fast mode"; clkspeed "Clock speed (kHz)"; timeout "Timeout (ms)"; writecount "Bytes write count"; readcount "Bytes read count"; sdapin "SDA pin"; sclpin "SCL pin"; waitwritetime "Wait write time (ms), default is 0"; inputtypearray "Input type array"; outputtypearray "Output type array"; confstr "Configuration string"; sampletime "Sample time (sec)"; sampletimestr "Compiled sample time (sec) in string"
      mask init:
      | stm32f4_i2c_callback('init');
      mask Help: web(fullfile(waijungdocroot,'stm32f4_i2c.htm'), '-browser')
      mask TypeOptions configuration: Setup | Transaction
      mask Callback configuration: stm32f4_i2c_callback('configuration');
      mask TypeOptions module: 1 | 2 | 3
      mask Callback module: stm32f4_i2c_callback('module');
      mask TypeOptions transfer: Blocking | Non-blocking
      mask TypeOptions dutycycle: TLow/THigh = 16/9 | TLow/THigh = 2
      mask Callback dutycycle: stm32f4_i2c_callback('dutycycle');
      mask Callback writecount: stm32f4_i2c_callback('writecount');
      mask Callback readcount: stm32f4_i2c_callback('readcount');
      mask TypeOptions sdapin: - | C9
      mask Callback sdapin: stm32f4_i2c_callback('sdapin');
      mask TypeOptions sclpin: - | A8
      mask Callback sclpin: stm32f4_i2c_callback('sclpin');
      mask Callback confstr: stm32f4_i2c_callback('confstr');
      mask Callback sampletime: stm32f4_i2c_callback('sampletime');
      mask Callback sampletimestr: stm32f4_i2c_callback('sampletimestr');
      mask Callback blockid: stm32f4_i2c_callback('blockid');
      mask Display: text(0.5, 0.5, 'Module: I2C1\nTransfer: Blocking\nWrite: 2 bytes\nRead: 0 bytes\nTs (sec): -1','ver','middle','hor','center');port_label('input', 1,'SlvAddr');port_label('input', 2,'Wr0 (uint8)');port_label('input', 3,'Wr1 (uint8)');port_label('output', 1,'Status');
  SlvAddr1 : Constant  Value=hex2dec('D2')  OutDataTypeStr=uint8  SampleTime=-1
  Subsystem : Subsystem
  Subsystem1 : Subsystem
  Terminator : Terminator
  wires:
  I2C Master Read/Write1/1 -> Compare To Zero1/1
  I2C Master Read/Write/1 -> Compare To Zero/1
  CNTRL_REG4/1 -> I2C Master Read/Write1/2
  FS 250/1 -> I2C Master Read/Write1/3
  Enable/1 -> I2C Master Read/Write/3
  CNTRL_REG1/1 -> I2C Master Read/Write/2
  SlvAddr1/1 -> I2C Master Read/Write1/1, I2C Master Read/Write/1
  Compare To Zero/1 -> Subsystem/Enable
  Compare To Zero1/1 -> Subsystem1/Enable
  Subsystem/1(Out1) -> Bitwise Operator/1
  Subsystem1/1(Out1) -> Bitwise Operator/2
  Bitwise Operator/1 -> Terminator/1

== system NE_Red_Rooster_Delta_B/Chart/spaceorient/Accelerometr/Manipulate Data ==
  LowAddress : Inport
  HighAddress : Inport  Port=2
  Add : Sum
  Data Type Conversion : DataTypeConversion  OutDataTypeStr=int16
  Data Type Conversion1 : DataTypeConversion  OutDataTypeStr=int16
  Shift Arithmetic1 : ArithShift  BitShiftNumber=8  BitShiftDirection=Left
  RawAccData : Outport
  wires:
  LowAddress/1 -> Data Type Conversion/1
  HighAddress/1 -> Data Type Conversion1/1
  Data Type Conversion/1 -> Add/1
  Data Type Conversion1/1 -> Shift Arithmetic1/1
  Shift Arithmetic1/1 -> Add/2
  Add/1 -> RawAccData/1

== system NE_Red_Rooster_Delta_B/Chart/spaceorient/Accelerometr/Manipulate Data1 ==
  LowAddress : Inport
  HighAddress : Inport  Port=2
  Add : Sum
  Data Type Conversion : DataTypeConversion  OutDataTypeStr=int16
  Data Type Conversion1 : DataTypeConversion  OutDataTypeStr=int16
  Shift Arithmetic1 : ArithShift  BitShiftNumber=8  BitShiftDirection=Left
  RawAccData : Outport
  wires:
  Add/1 -> RawAccData/1
  Shift Arithmetic1/1 -> Add/2
  Data Type Conversion1/1 -> Shift Arithmetic1/1
  Data Type Conversion/1 -> Add/1
  HighAddress/1 -> Data Type Conversion1/1
  LowAddress/1 -> Data Type Conversion/1

== system NE_Red_Rooster_Delta_B/Chart/spaceorient/Accelerometr/Manipulate Data2 ==
  LowAddress : Inport
  HighAddress : Inport  Port=2
  Add : Sum
  Data Type Conversion : DataTypeConversion  OutDataTypeStr=int16
  Data Type Conversion1 : DataTypeConversion  OutDataTypeStr=int16
  Shift Arithmetic1 : ArithShift  BitShiftNumber=8  BitShiftDirection=Left
  RawAccData : Outport
  wires:
  LowAddress/1 -> Data Type Conversion/1
  HighAddress/1 -> Data Type Conversion1/1
  Data Type Conversion/1 -> Add/1
  Data Type Conversion1/1 -> Shift Arithmetic1/1
  Shift Arithmetic1/1 -> Add/2
  Add/1 -> RawAccData/1

== system NE_Red_Rooster_Delta_B/Chart/spaceorient/Accelerometr/Subsystem ==
  Enable : EnablePort
  Logical Operator : Logic  Operator=NOT  AllPortsSameDT=off  OutDataTypeStr=boolean
  Memory : Memory  InheritSampleTime=on
  Out1 : Outport
  wires:
  Logical Operator/1 -> Out1/1, Memory/1
  Memory/1 -> Logical Operator/1

== system NE_Red_Rooster_Delta_B/Chart/spaceorient/Accelerometr/Subsystem1 ==
  Enable : EnablePort
  Logical Operator : Logic  Operator=NOT  AllPortsSameDT=off  OutDataTypeStr=boolean
  Memory : Memory  InheritSampleTime=on
  Out1 : Outport
  wires:
  Memory/1 -> Logical Operator/1
  Logical Operator/1 -> Memory/1, Out1/1

== system NE_Red_Rooster_Delta_B/Chart/spaceorient/Accelerometr/Subsystem2 ==
  Enable : EnablePort
  Logical Operator : Logic  Operator=NOT  AllPortsSameDT=off  OutDataTypeStr=boolean
  Memory : Memory  InheritSampleTime=on
  Out1 : Outport
  wires:
  Logical Operator/1 -> Out1/1, Memory/1
  Memory/1 -> Logical Operator/1

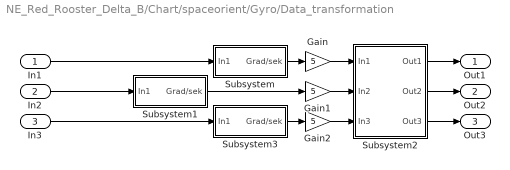
== system NE_Red_Rooster_Delta_B/Chart/spaceorient/Gyro/Data_transformation ==
  In1 : Inport
  In2 : Inport  Port=2
  In3 : Inport  Port=3
  Gain : Gain  Gain=5
  Gain1 : Gain  Gain=5
  Gain2 : Gain  Gain=5
  Subsystem : Subsystem
  Subsystem1 : Subsystem
  Subsystem2 : Subsystem
  Subsystem3 : Subsystem
  Out1 : Outport
  Out2 : Outport  Port=2
  Out3 : Outport  Port=3
  wires:
  Subsystem2/1(Out1) -> Out1/1
  Subsystem2/2(Out2) -> Out2/1
  Subsystem2/3(Out3) -> Out3/1
  In1/1 -> Subsystem/1(In1)
  In2/1 -> Subsystem1/1(In1)
  In3/1 -> Subsystem3/1(In1)
  Subsystem/1(Grad/sek) -> Gain/1
  Subsystem1/1(Grad/sek) -> Gain1/1
  Subsystem3/1(Grad/sek) -> Gain2/1
  Gain/1 -> Subsystem2/1(In1)
  Gain1/1 -> Subsystem2/2(In2)
  Gain2/1 -> Subsystem2/3(In3)

== system NE_Red_Rooster_Delta_B/Chart/spaceorient/Gyro/L3G4200D ==
  Read L3G4200D : Subsystem  TreatAsAtomicUnit=on
  SlvAddr1 : Constant  Value=hex2dec('D2')  OutDataTypeStr=uint8  SampleTime=-1
  Status : Outport
  X : Outport  Port=2
  Y : Outport  Port=3
  Z : Outport  Port=4
  wires:
  Read L3G4200D/4(OUT_Z) -> Z/1
  Read L3G4200D/3(OUT_Y) -> Y/1
  Read L3G4200D/2(OUT_X) -> X/1
  Read L3G4200D/1(Status) -> Status/1
  SlvAddr1/1 -> Read L3G4200D/1(SlvAddr)

== system NE_Red_Rooster_Delta_B/Chart/spaceorient/Gyro/Success ==
  In1 : Inport
  In2 : Inport  Port=2
  In3 : Inport  Port=3
  Enable : EnablePort  PropagateVarSize=During execution
  Data Type Conversion : DataTypeConversion  OutDataTypeStr=int16
  Demux : Demux  Outputs=3
  Gain : Gain  Gain=250/2^15  ParamDataTypeStr=single  OutDataTypeStr=single
  Mux : Mux  Inputs=3
  Gyr_X : Outport
  Gyr_Y : Outport  Port=2
  Gyr_Z : Outport  Port=3
  wires:
  Data Type Conversion/1 -> Gain/1
  In3/1 -> Mux/3
  In2/1 -> Mux/2
  In1/1 -> Mux/1
  Demux/3 -> Gyr_Z/1
  Demux/2 -> Gyr_Y/1
  Demux/1 -> Gyr_X/1
  Gain/1 -> Demux/1
  Mux/1 -> Data Type Conversion/1

== system NE_Red_Rooster_Delta_B/Chart/initgyro/Init_L3GD4200 /Init L3G4200D/Subsystem ==
  Enable : EnablePort
  Logical Operator : Logic  Operator=NOT  AllPortsSameDT=off  OutDataTypeStr=boolean
  Memory : Memory  InheritSampleTime=on
  Out1 : Outport
  wires:
  Logical Operator/1 -> Out1/1, Memory/1
  Memory/1 -> Logical Operator/1

== system NE_Red_Rooster_Delta_B/Chart/initgyro/Init_L3GD4200 /Init L3G4200D/Subsystem1 ==
  Enable : EnablePort
  Logical Operator : Logic  Operator=NOT  AllPortsSameDT=off  OutDataTypeStr=boolean
  Memory : Memory  InheritSampleTime=on
  Out1 : Outport
  wires:
  Memory/1 -> Logical Operator/1
  Logical Operator/1 -> Memory/1, Out1/1

== system NE_Red_Rooster_Delta_B/Chart/spaceorient/Gyro/Data_transformation/Subsystem ==
  In1 : Inport
  Constant : Constant  Value=17.5
  Constant1 : Constant  Value=1000
  Divide : Product  Inputs=*/
  Product : Product
  Grad/sek : Outport
  wires:
  Constant1/1 -> Divide/2
  Product/1 -> Divide/1
  Constant/1 -> Product/2
  In1/1 -> Product/1
  Divide/1 -> Grad/sek/1

== system NE_Red_Rooster_Delta_B/Chart/spaceorient/Gyro/Data_transformation/Subsystem1 ==
  In1 : Inport
  Constant : Constant  Value=17.5
  Constant1 : Constant  Value=1000
  Divide : Product  Inputs=*/
  Product : Product
  Grad/sek : Outport
  wires:
  Divide/1 -> Grad/sek/1
  In1/1 -> Product/1
  Constant/1 -> Product/2
  Product/1 -> Divide/1
  Constant1/1 -> Divide/2

== system NE_Red_Rooster_Delta_B/Chart/spaceorient/Gyro/Data_transformation/Subsystem2 ==
  In1 : Inport
  In2 : Inport  Port=2
  In3 : Inport  Port=3
  Data Type Conversion : DataTypeConversion  OutDataTypeStr=single
  Data Type Conversion1 : DataTypeConversion  OutDataTypeStr=single
  Data Type Conversion2 : DataTypeConversion  OutDataTypeStr=single
  From_free_data_to_Angle : Subsystem
  Out1 : Outport
  Out2 : Outport  Port=2
  Out3 : Outport  Port=3
  wires:
  In1/1 -> From_free_data_to_Angle/3(W_Roll)
  From_free_data_to_Angle/1(Angle_Yaw) -> Data Type Conversion2/1
  From_free_data_to_Angle/2(Angle_Pitch) -> Data Type Conversion1/1
  From_free_data_to_Angle/3(Angle_Roll) -> Data Type Conversion/1
  In2/1 -> From_free_data_to_Angle/2(W_Pitch)
  In3/1 -> From_free_data_to_Angle/1(W_Yaw)
  Data Type Conversion/1 -> Out3/1
  Data Type Conversion1/1 -> Out2/1
  Data Type Conversion2/1 -> Out1/1

== system NE_Red_Rooster_Delta_B/Chart/spaceorient/Gyro/Data_transformation/Subsystem3 ==
  In1 : Inport
  Constant : Constant  Value=17.5
  Constant1 : Constant  Value=1000
  Divide : Product  Inputs=*/
  Product : Product
  Grad/sek : Outport
  wires:
  Constant1/1 -> Divide/2
  Product/1 -> Divide/1
  Constant/1 -> Product/2
  In1/1 -> Product/1
  Divide/1 -> Grad/sek/1
